simulink model "ultracap_converter_simplified_PI_control_v5"  (R2015a)
settings: Solver=ode45  StartTime=0.0  StopTime=0.6  FixedStep=TsampleSimulink  MaxStep=1e-6  RelTol=1e-3
values from neighbouring files (symbols this model uses):
  Ea = 4.2622    [me547_based_PI_controller_v3.m]
  Ra = 0.0560    (= 0.056)    [me547_based_PI_controller_v3.m]
  tf_TWA = tf([Ts 0], [1 -1], Ts)    [me547_based_PI_controller_v3.m]
  Ts = 1/fs    (= 0.0002)    [load_system_parameters.m]
  Vbat = 48    [load_system_parameters.m]
undefined symbols (not defined in the file or in its folder): fdesignblkfcn, gcbh, ILcommand_z, plecs
libraries: dspsigops x2, dspstat3 x1, simulink x1
settings Model: Creator=Raghav  LastModifiedBy=Anantharaghavan
settings OptimizationCC: ExpressionDepthLimit=2147483647
settings DebuggingCC: UnderspecifiedInitializationDetection=Classic  MergeDetectMultiDrivingBlocksExec=none  SolverPrmCheckMsg=warning  StateNameClashWarn=warning

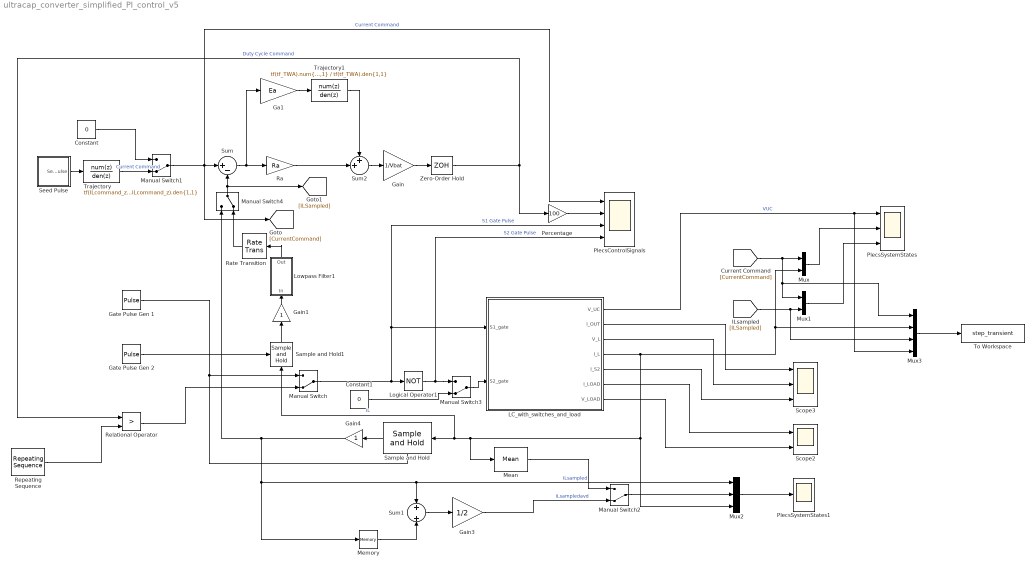
== system ultracap_converter_simplified_PI_control_v5 ==
  Constant : Constant  Value=0
  Constant1 : Constant  Value=0
  Ga1 : Gain  Gain=Ea  SampleTime=Ts
  Gain : Gain  Gain=1/Vbat
  Gain1 : Gain  SampleTime=Ts/10
  Gain3 : Gain  Gain=1/2
  Gain4 : Gain  SampleTime=Ts
  Gate Pulse Gen 1 : DiscretePulseGenerator  PulseType=Time based  Period=Ts  PulseWidth=71.42
  Gate Pulse Gen 2 : DiscretePulseGenerator  PulseType=Time based  Period=Ts/10  PulseWidth=71.42
  LC_with_switches_and_load : Subsystem  LoadFcn=plecs('sl', 200);  InitFcn=plecs('sl', 214);  StartFcn=plecs('sl', 208);  StopFcn=plecs('sl', 209);  mask(PlecsCircuit){PLECSData=<binary blob, 2400 chars, not shown>}
      mask prompts: PLECSData "PLECS Data (Do not delete or modify!)"
      mask init:
      | % PLACE CUSTOM INITIALIZATIONS ABOVE
      | % DO NOT REMOVE
      | plecs('sl', 215);
      | % DO NOT REMOVE
      settings: CopyFcn=plecs('sl', 203);  DeleteFcn=plecs('sl', 205);  UndoDeleteFcn=plecs('sl', 206);  PreSaveFcn=plecs('sl', 211);  PostSaveFcn=plecs('sl', 201);  NameChangeFcn=plecs('sl', 210);  DestroyFcn=plecs('sl', 207);  PreCopyFcn=plecs('sl', 216);  OpenFcn=plecs('sl', 202);  ErrorFcn=plerrorfcn
      mask Help: web(['file:///' fullfile(plecsdoc, 'creatingacircuit.html')])
      mask Display: disp('PLECS\nCircuit')
  Logical Operator1 : Logic  Operator=NOT  AllPortsSameDT=off  OutDataTypeStr=boolean
  Lowpass Filter1 : Subsystem  DialogController=fdesignblkfcn  InitFcn=fdesignblkfcn(gcbh, {'InitFcn'});  mask(Lowpass Filter){}
      mask help: Design a lowpass filter
      settings: CopyFcn=fdesignblkfcn(gcbh, {'CopyFcn'});
      mask Help: helpview(mapfilelocation('dsp'), 'dsplowpassfilter');
      mask Display: disp('Lowpass')
  Manual Switch{,1..4} (5 alike) : ManualSwitch  CurrentSetting=0
  Mean : dspstat3/Mean  run=off  reset_popup=None  InputProcessing=Columns as channels (frame based)  directionMode=Each column  dimension=1  treatSBRowAsCol=off  roiEnable=off  roiType=Rectangles  roiPortion=Entire ROI  roiOutput=Individual statistics for each ROI  roiFlag=off  outputDataTypeStr=Inherit: Same as accumulator  outputLastDataTypeStr=Inherit: Same as accumulator  outputMin=[]  outputMax=[]  roundingMode=Floor  overflowMode=off
  Memory : Memory  InheritSampleTime=on  LinearizeMemory=on  LinearizeAsDelay=on
  Mux : Mux  Inputs=2
  Mux1 : Mux  Inputs=2
  Mux2 : Mux  Inputs=3
  Mux3 : Mux
  Percentage : Gain  Gain=100
  PlecsControlSignals : Scope  NumInputPorts=4
      settings: YMin=0~0~-0.5~-0.5  YMax=5~1~1.5~1.5  SaveName=PlecsControlSignals
  PlecsSystemStates : Scope  NumInputPorts=3
      settings: ShowLegends=on  YMin=14.9875~8~8.7  YMax=14.9905~23~10  SaveName=PlecsSystemStates
  PlecsSystemStates1 : Scope
      settings: ShowLegends=on  YMin=0  YMax=10.5  SaveName=PlecsSystemStates1
  Ra : Gain  Gain=Ra  SampleTime=Ts
  Rate Transition : RateTransition  OutPortSampleTime=Ts
  Relational Operator : RelationalOperator  Priority=50  Operator=>  OutDataTypeStr=boolean
  Repeating Sequence : simulink/Sources/Repeating Sequence  rep_seq_t=[0 Ts]  rep_seq_y=[0 1]
  Sample and Hold : dspsigops/Sample and Hold  trig=Rising edge  initCond=0  latchinput=on
  Sample and Hold1 : dspsigops/Sample and Hold  trig=Rising edge  initCond=0  latchinput=on
  Scope2 : Scope  NumInputPorts=2
      settings: ShowLegends=on  YMin=-5~-5  YMax=5~5  SaveName=ScopeData2
  Scope3 : Scope  NumInputPorts=3
      settings: ShowLegends=on  YMin=0~-50~-5  YMax=3.75~650~5  SaveName=Scope3
  Seed Pulse : Subsystem
  Sum : Sum  Inputs=|+-
  Sum1 : Sum  Inputs=+|+
  Sum2 : Sum  Inputs=++|
  To Workspace : ToWorkspace  VariableName=step_transient  SaveFormat=Structure With Time  SampleTime=-1
  Trajectory : DiscreteTransferFcn  Numerator=tf(ILcommand_z).num{1,1}  Denominator=tf(ILcommand_z).den{1,1}  SampleTime=Ts
  Trajectory1 : DiscreteTransferFcn  Numerator=tf(tf_TWA).num{1,1}  Denominator=tf(tf_TWA).den{1,1}  SampleTime=Ts
  Zero-Order Hold : ZeroOrderHold  SampleTime=Ts
  wires:
  LC_with_switches_and_load/1(V_UC) -> Mux3/4, PlecsSystemStates/1  "VUC"
  LC_with_switches_and_load/7(V_LOAD) -> Scope2/2
  LC_with_switches_and_load/4(I_L) -> Mux3/2, Mux/2, Mux2/3, Mean/1, Sample and Hold1/1, Sample and Hold/1  "IL"
  LC_with_switches_and_load/6(I_LOAD) -> Scope2/1
  Logical Operator1/1 -> Manual Switch3/1, PlecsControlSignals/4  "S2 Gate Pulse"
  Manual Switch/1 -> LC_with_switches_and_load/1(S1_gate), PlecsControlSignals/3, Logical Operator1/1  "S1 Gate Pulse"
  Seed Pulse/1(Seed Pulse) -> Trajectory/1
  Manual Switch1/1 -> PlecsControlSignals/1, [CurrentCommand], Sum/1  "Current Command"
  Sum/1 -> Ga1/1, Ra/1
  Ra/1 -> Sum2/2
  Zero-Order Hold/1 -> Relational Operator/1, Percentage/1  "Duty Cycle Command"
  Repeating Sequence/1 -> Relational Operator/2
  Gain/1 -> Zero-Order Hold/1
  Gate Pulse Gen 1/1 -> Sample and Hold/Trigger, Manual Switch/1
  Relational Operator/1 -> Manual Switch/2
  Memory/1 -> Sum1/2
  Sum1/1 -> Gain3/1
  Mux2/1 -> PlecsSystemStates1/1
  Sample and Hold/1 -> Gain4/1
  Gain4/1 -> Manual Switch4/1, Sum1/1, Mux2/1, Memory/1  "ILsampled"
  Gain3/1 -> Manual Switch2/2  "ILsampledavd"
  Mean/1 -> Manual Switch2/1
  Manual Switch2/1 -> Mux2/2
  LC_with_switches_and_load/2(I_OUT) -> Scope3/1
  LC_with_switches_and_load/3(V_L) -> Scope3/2
  LC_with_switches_and_load/5(I_S2) -> Scope3/3
  [CurrentCommand] -> Mux3/1, Mux1/1, Mux/1
  Mux/1 -> PlecsSystemStates/2
  Mux1/1 -> PlecsSystemStates/3
  [ILSampled] -> Mux3/3, Mux1/2
  Percentage/1 -> PlecsControlSignals/2
  Sum2/1 -> Gain/1
  Trajectory1/1 -> Sum2/1
  Ga1/1 -> Trajectory1/1
  Trajectory/1 -> Manual Switch1/2  "Current Command"
  Constant/1 -> Manual Switch1/1
  Manual Switch3/1 -> LC_with_switches_and_load/2(S2_gate)
  Constant1/1 -> Manual Switch3/2
  Lowpass Filter1/1(Out) -> Rate Transition/1
  Sample and Hold1/1 -> Gain1/1
  Gate Pulse Gen 2/1 -> Sample and Hold1/Trigger
  Gain1/1 -> Lowpass Filter1/1(In)
  Rate Transition/1 -> Manual Switch4/2
  Manual Switch4/1 -> [ILSampled], Sum/2
  Mux3/1 -> To Workspace/1

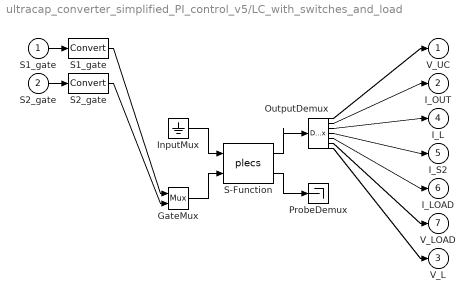
== system ultracap_converter_simplified_PI_control_v5/LC_with_switches_and_load ==
  S1_gate : Inport  PortDimensions=1
  S2_gate : Inport  Port=2  PortDimensions=1
  " GateMux " : Mux  Inputs=[ 1 1 ]
  " InputMux " : Ground
  " OutputDemux " : Demux  Outputs=[ 1 1 1 1 1 1 1 ]
  " ProbeDemux " : Terminator
  " S-Function " : S-Function  FunctionName=plecs
  " S1_gate " : DataTypeConversion  SaturateOnIntegerOverflow=on  RndMeth=Zero
  " S2_gate " : DataTypeConversion  SaturateOnIntegerOverflow=on  RndMeth=Zero
  V_UC : Outport  PortDimensions=1
  I_OUT : Outport  Port=2  PortDimensions=1
  V_L : Outport  Port=3  PortDimensions=1
  I_L : Outport  Port=4  PortDimensions=1
  I_S2 : Outport  Port=5  PortDimensions=1
  I_LOAD : Outport  Port=6  PortDimensions=1
  V_LOAD : Outport  Port=7  PortDimensions=1
  wires:
  " S-Function "/2 -> " ProbeDemux "/1
  " GateMux "/1 -> " S-Function "/2
  " InputMux "/1 -> " S-Function "/1
  " S-Function "/1 -> " OutputDemux "/1
  S1_gate/1 -> " S1_gate "/1
  " S1_gate "/1 -> " GateMux "/1
  S2_gate/1 -> " S2_gate "/1
  " S2_gate "/1 -> " GateMux "/2
  " OutputDemux "/1 -> V_UC/1
  " OutputDemux "/2 -> I_OUT/1
  " OutputDemux "/3 -> I_L/1
  " OutputDemux "/4 -> I_S2/1
  " OutputDemux "/5 -> I_LOAD/1
  " OutputDemux "/6 -> V_LOAD/1
  " OutputDemux "/7 -> V_L/1

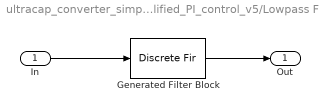
== system ultracap_converter_simplified_PI_control_v5/Lowpass Filter1 ==
  In : Inport
  Generated Filter Block : DiscreteFir  Tag=BlockMethodSubSystem  Coefficients=[6.0803750441260938e-05 -0.000218444594793199 0.00058289284039042349 -0.0013049955363826512 0.0025992795839228358 -0.0047526300439456031 0.0081373750217281545 -0.013236499174731804 0.020702325169230491 -0.031500650120221838 0.047280292569303259 -0.071419893070525098 0.11263745297952366 -0.20308297923388002 0.6335249405004364 0.6335249405004364 -0.20308297923388002 0.11263745297952366 -0.071419893070525098 0.047280292569303259 -0.031500650120221838 0.020702325169230491 -0.013236499174731804 0.0081373750217281545 -0.0047526300439456031 0.0025992795839228358 -0.0013049955363826512 0.00058289284039042349 -0.000218444594793199 6.0803750441260938e-05]  InputProcessing=Columns as channels (frame based)
  Out : Outport
  wires:
  Generated Filter Block/1 -> Out/1
  In/1 -> Generated Filter Block/1

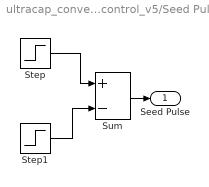
== system ultracap_converter_simplified_PI_control_v5/Seed Pulse ==
  Step : Step  Time=10*Ts  SampleTime=0
  Step1 : Step  Time=10*Ts+Ts/2  SampleTime=0
  Sum : Sum  Inputs=+-
  Seed Pulse : Outport
  wires:
  Sum/1 -> Seed Pulse/1
  Step/1 -> Sum/1
  Step1/1 -> Sum/2
